simulink model "motor"  (R2015a)
settings: Solver=ode45  StartTime=0.0  StopTime=10.0  RelTol=1e-3
undefined symbols (not defined in the file): f, J, k, La, Ra
libraries: powerlib x1
settings Model: Creator=Yaman  LastModifiedBy=MBK

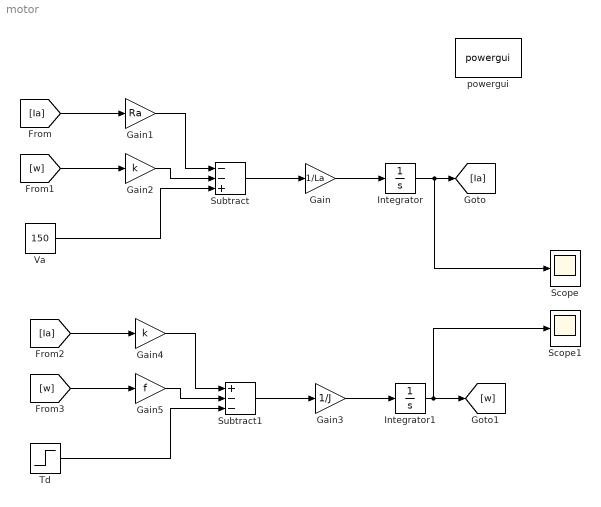
== system motor ==
  Gain : Gain  Gain=1/La
  Gain1 : Gain  Gain=Ra
  Gain2 : Gain  Gain=k
  Gain3 : Gain  Gain=1/J
  Gain4 : Gain  Gain=k
  Gain5 : Gain  Gain=f
  Integrator : Integrator
  Integrator1 : Integrator
  Scope : Scope
  Scope1 : Scope
  Subtract : Sum  Inputs=--+
  Subtract1 : Sum  Inputs=+--
  Td : Step  Time=5  SampleTime=1.2
  "Va " : Constant  Value=150
  powergui : powerlib/powergui  Priority=1  SimulationMode=Continuous  SolverType=Tustin/Backward Euler (TBE)  SampleTime=50e-6  frequency=60  SPID=off  DisableSnubberDevices=off  DisableRonSwitches=off  DisableVfSwitches=off  SwTol=0  DisplayEquations=off  Interpol=off  methode=off  Ts=100  FunctionMessages=off  echomessages=off  HookPort=off  EnableUseOfTLC=off  x0status=blocks  frequencyindice=60  Pbase=100e6  ErrMax=1e-4  Iterations=50  UnitsV=kV  UnitsW=MW  buscounter=0  RestoreLinks=warning  ResistiveCurrentMeasurement=off  Frange=[0:2:500]  Ylog=off  Xlog=on  ShowGrid=off  save=off  variable=ZData  structure=0  ZoomFFT=off  StartTime=0.0  cycles=1  DisplayStyle=1  fundamental=60  FreqAxis=off  MaxFrequency=1000  frequencyindicesteady=1  RmsSteady=1  display=off
  wires:
  "Va "/1 -> Subtract/3
  Subtract/1 -> Gain/1
  Gain/1 -> Integrator/1
  Integrator/1 -> Scope/1, [Ia]
  [w] -> Gain2/1
  [Ia] -> Gain1/1
  Gain1/1 -> Subtract/1
  Gain2/1 -> Subtract/2
  Td/1 -> Subtract1/3
  Subtract1/1 -> Gain3/1
  Integrator1/1 -> Scope1/1, [w]
  [w] -> Gain5/1
  [Ia] -> Gain4/1
  Gain4/1 -> Subtract1/1
  Gain5/1 -> Subtract1/2
  Gain3/1 -> Integrator1/1
